simulink model "n_metro"  (Simulink 6.6)
settings: Solver=ode45  StartTime=0.0  StopTime=L  RelTol=1e-6
undefined symbols (not defined in the file): D, Delta, DiscIntNeverNeededParam, dpmax, K, Ka, Kdn, Ki, Kv, L, M_ecart, N, Tau, Td, Te, Tm, Tstart, Tstop
settings Model: Creator=admin  LastModifiedBy=acco
settings DataIOCC: SignalLoggingName=sigsOut
settings DebuggingCC: SignalResolutionControl=TryResolveAllWithWarning  SolverPrmCheckMsg=none  MultiTaskDSMMsg=warning  MultiTaskCondExecSysMsg=none  StrictBusMsg=None
settings HardwareCC: TargetUnknown=on
settings RTWCC: IncludeERTFirstTime=on

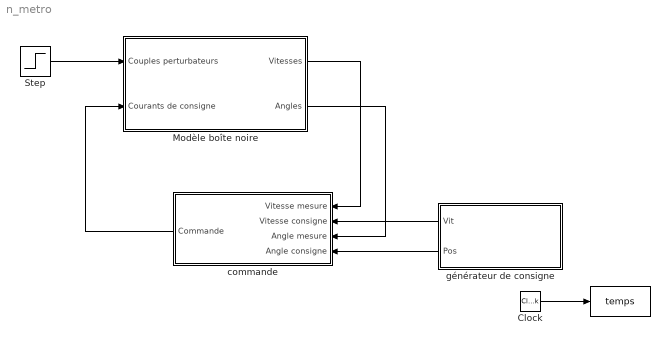
== system n_metro ==
  " " : ToWorkspace  VariableName=temps  SampleTime=-1  SaveFormat=Array
  Clock : DigitalClock  SampleTime=Te
  Modèle boîte noire : Subsystem
  Step : Step  Time=L*0.1  Before=zeros(N,1)  After=-ones(N,1)*0  SampleTime=Te
  commande : Subsystem  Orientation=left  TreatAsAtomicUnit=on
      settings: RTWSystemCode=Function  RTWFcnNameOpts=Use subsystem name  RTWFileNameOpts=Use subsystem name
  générateur de consigne : Subsystem  Orientation=left
  wires:
  Step/1 -> Modèle boîte noire/1(Couples perturbateurs)
  Modèle boîte noire/2(Angles) -> commande/3(Angle mesure)
  Clock/1 -> " "/1
  commande/1(Commande) -> Modèle boîte noire/2(Courants de consigne)
  Modèle boîte noire/1(Vitesses) -> commande/1(Vitesse mesure)
  générateur de consigne/2(Pos) -> commande/4(Angle consigne)
  générateur de consigne/1(Vit) -> commande/2(Vitesse consigne)

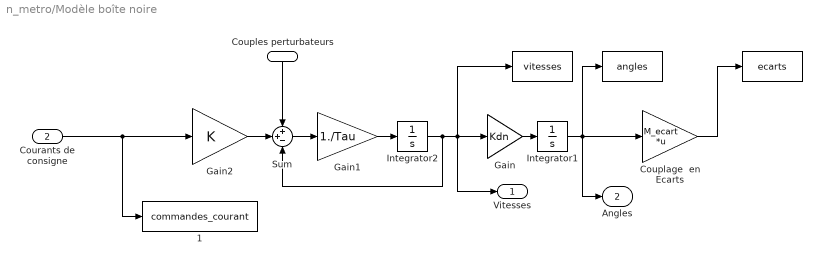
== system n_metro/Modèle boîte noire ==
  Couples perturbateurs : Inport  Orientation=down
  Courants de consigne : Inport  Port=2
  " " : ToWorkspace  VariableName=vitesses  SampleTime=Te  SaveFormat=Array
  "  " : ToWorkspace  VariableName=angles  SampleTime=Te  SaveFormat=Array
  "   " : ToWorkspace  VariableName=ecarts  SampleTime=Te  SaveFormat=Array
  "   1" : ToWorkspace  VariableName=commandes_courant  SampleTime=-1  SaveFormat=Array
  Couplage  en Ecarts : Gain  Gain=M_ecart  Multiplication=Matrix(K*u)  SaturateOnIntegerOverflow=on
  Gain : Gain  Gain=Kdn
  Gain1 : Gain  Gain=1./Tau
  Gain2 : Gain  Gain=K
  Integrator1 : Integrator  InitialCondition=[0:N-1]'*Delta
  Integrator2 : Integrator  InitialCondition=zeros(N,1)
  Sum : Sum  Inputs=++-  SaturateOnIntegerOverflow=on
  Vitesses : Outport
  Angles : Outport  Port=2
  wires:
  Couplage  en Ecarts/1 -> "   "/1
  Courants de consigne/1 -> "   1"/1, Gain2/1
  Couples perturbateurs/1 -> Sum/1
  Gain/1 -> Integrator1/1
  Sum/1 -> Gain1/1
  Integrator2/1 -> " "/1, Vitesses/1, Gain/1, Sum/3
  Integrator1/1 -> Couplage  en Ecarts/1, Angles/1, "  "/1
  Gain1/1 -> Integrator2/1
  Gain2/1 -> Sum/2

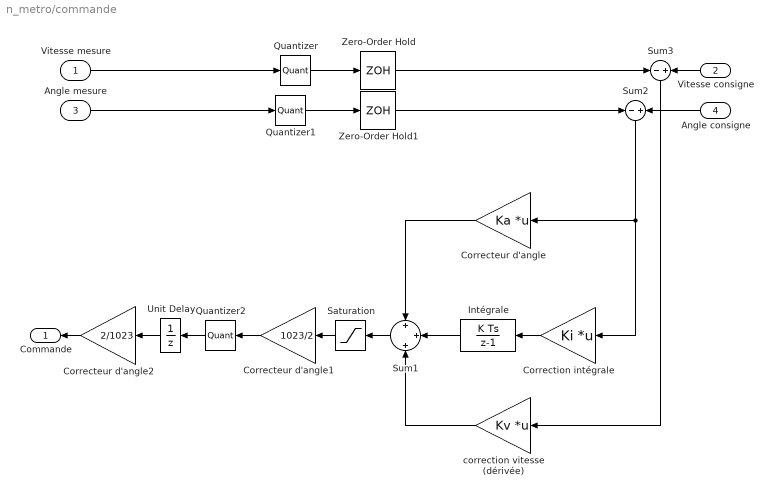
== system n_metro/commande ==
  Vitesse mesure : Inport
  Vitesse consigne : Inport  Orientation=left  Port=2
  Angle mesure : Inport  Port=3
  Angle consigne : Inport  Orientation=left  Port=4
  Correcteur d'angle : Gain  Orientation=left  Gain=Ka  Multiplication=Matrix(K*u)  SaturateOnIntegerOverflow=on
  Correcteur d'angle1 : Gain  Orientation=left  Gain=1023/2  SaturateOnIntegerOverflow=on
  Correcteur d'angle2 : Gain  Orientation=left  Gain=2/1023  SaturateOnIntegerOverflow=on
  Correction intégrale : Gain  Orientation=left  Gain=Ki  Multiplication=Matrix(K*u)  SaturateOnIntegerOverflow=on
  Intégrale : DiscreteIntegrator  Orientation=left  InitialCondition=zeros(N,1)  SampleTime=Te  LimitOutput=on  UpperSaturationLimit=1  LowerSaturationLimit=-1  ICPrevOutput=DiscIntNeverNeededParam  ICPrevScaledInput=DiscIntNeverNeededParam
  Quantizer : Quantizer  QuantizationInterval=1
  Quantizer1 : Quantizer  QuantizationInterval=1
  Quantizer2 : Quantizer  Orientation=left  QuantizationInterval=1
  Saturation : Saturate  Orientation=left  UpperLimit=1  LowerLimit=-1
  Sum1 : Sum  Orientation=left  Inputs=+|+|+  SaturateOnIntegerOverflow=on
  Sum2 : Sum  Orientation=down  Inputs=-|+  SaturateOnIntegerOverflow=on
  Sum3 : Sum  Orientation=down  Inputs=-|+  SaturateOnIntegerOverflow=on
  Unit Delay : UnitDelay  Orientation=left  SampleTime=Te
  Zero-Order Hold : ZeroOrderHold  SampleTime=Te
  Zero-Order Hold1 : ZeroOrderHold  SampleTime=Te
  correction vitesse (dérivée) : Gain  Orientation=left  Gain=Kv  Multiplication=Matrix(K*u)  SaturateOnIntegerOverflow=on
  Commande : Outport  Orientation=left
  wires:
  Sum2/1 -> Correcteur d'angle/1, Correction intégrale/1
  Correcteur d'angle/1 -> Sum1/1
  Sum3/1 -> correction vitesse (dérivée)/1
  correction vitesse (dérivée)/1 -> Sum1/3
  Correction intégrale/1 -> Intégrale/1
  Vitesse consigne/1 -> Sum3/2
  Angle consigne/1 -> Sum2/2
  Vitesse mesure/1 -> Quantizer/1
  Angle mesure/1 -> Quantizer1/1
  Sum1/1 -> Saturation/1
  Zero-Order Hold/1 -> Sum3/1
  Zero-Order Hold1/1 -> Sum2/1
  Quantizer/1 -> Zero-Order Hold/1
  Quantizer1/1 -> Zero-Order Hold1/1
  Intégrale/1 -> Sum1/2
  Saturation/1 -> Correcteur d'angle1/1
  Correcteur d'angle1/1 -> Quantizer2/1
  Quantizer2/1 -> Unit Delay/1
  Unit Delay/1 -> Correcteur d'angle2/1
  Correcteur d'angle2/1 -> Commande/1

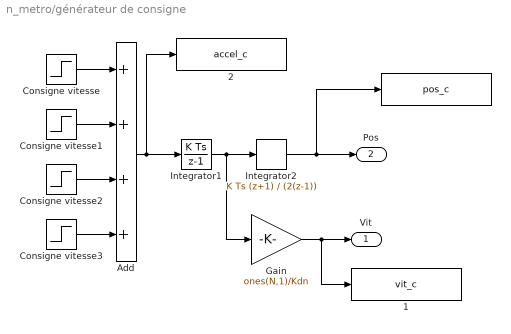
== system n_metro/générateur de consigne ==
  "  " : ToWorkspace  VariableName=pos_c  SampleTime=-1  SaveFormat=Array
  "  1" : ToWorkspace  VariableName=vit_c  SampleTime=-1  SaveFormat=Array
  "  2" : ToWorkspace  VariableName=accel_c  SampleTime=-1  SaveFormat=Array
  Add : Sum  Inputs=++++  OutScaling=2^-10
  Consigne vitesse : Step  Time=Tstart  After=dpmax/Tm  SampleTime=Te
  Consigne vitesse1 : Step  Time=Tstart+Tm  After=-dpmax/Tm  SampleTime=Te
  Consigne vitesse2 : Step  Time=Tstart+Tm+D  After=-dpmax/Td  SampleTime=Te
  Consigne vitesse3 : Step  Time=Tstop  After=dpmax/Td  SampleTime=Te
  Gain : Gain  Gain=ones(N,1)/Kdn
  Integrator1 : DiscreteIntegrator  gainval=1  SampleTime=Te  ICPrevOutput=DiscIntNeverNeededParam  ICPrevScaledInput=DiscIntNeverNeededParam
  Integrator2 : DiscreteIntegrator  IntegratorMethod=Integration: Trapezoidal  gainval=1  InitialCondition=[0:N-1]'*Delta  SampleTime=Te  ICPrevOutput=DiscIntNeverNeededParam  ICPrevScaledInput=DiscIntNeverNeededParam
  Vit : Outport
  Pos : Outport  Port=2
  wires:
  Consigne vitesse/1 -> Add/1
  Consigne vitesse1/1 -> Add/2
  Consigne vitesse2/1 -> Add/3
  Consigne vitesse3/1 -> Add/4
  Add/1 -> Integrator1/1, "  2"/1
  Integrator1/1 -> Integrator2/1, Gain/1
  Integrator2/1 -> Pos/1, "  "/1
  Gain/1 -> Vit/1, "  1"/1
